simulink model "allen_var_test"  (R2018b)
settings: Solver=FixedStepAuto  StartTime=0.0  StopTime=10.0  FixedStep=simParams.sample_time_s  RelTol=1e-3
undefined symbols (not defined in the file or in its folder): fswParams, gyroscope_lib, simParams
libraries: simulink x3
settings Model: Creator=Taylor  LastModifiedBy=Taylor

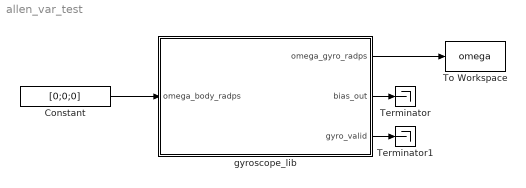
== system allen_var_test ==
  Constant : Constant  Value=[0;0;0]
  Terminator : Terminator
  Terminator1 : Terminator
  To Workspace : ToWorkspace  VariableName=omega  SampleTime=-1
      settings: Save2DSignal=2-D array (concatenate along first dimension)
  gyroscope_lib : Subsystem  AncestorBlock=gyroscope_lib/gyroscope_lib  mask{id_s=1}
      mask prompts: id_s "Choose the sensor ID"
      mask TypeOptions id_s: 1 | 2 | 3
      mask DialogControl DescGroupVar Prompt: SOC-i Gyroscope Model
      mask DialogControl DescTextVar Prompt: The spacecraft has three Bosch BMI055 gyroscopes.
  wires:
  Constant/1 -> gyroscope_lib/1(omega_body_radps)
  gyroscope_lib/1(omega_gyro_radps) -> To Workspace/1
  gyroscope_lib/2(bias_out) -> Terminator/1
  gyroscope_lib/3(gyro_valid) -> Terminator1/1

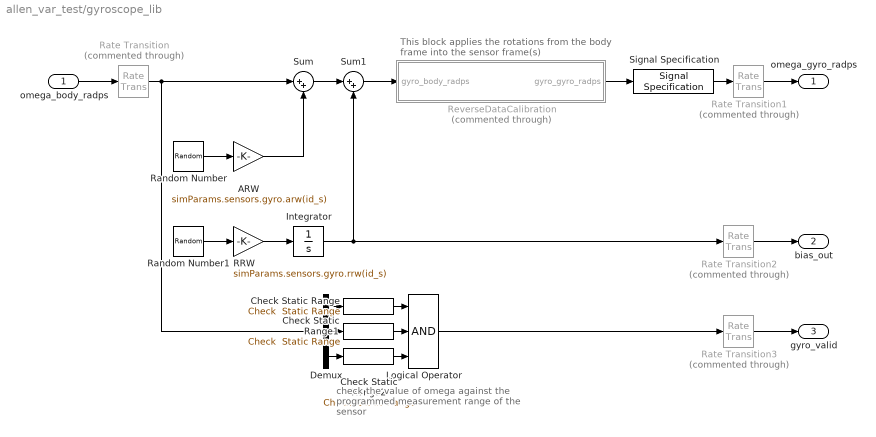
== system allen_var_test/gyroscope_lib ==
  note: check the value of omega against
      | the programmed measurement range
      | of the sensor
  note: This block applies the rotations from the
      | body frame into the sensor frame(s)
  omega_body_radps : Inport
  ARW : Gain  Gain=simParams.sensors.gyro.arw(id_s)
  Check Static Range : simulink/Model Verification/Check  Static Range  Description=simParams.sensors.gyro.w_min(id_s) <= u <= simParams.sensors.gyro.w_max(id_s)  max=simParams.sensors.gyro.w_max(id_s)  max_included=on  min=simParams.sensors.gyro.w_min(id_s)  min_included=on  enabled=on  stopWhenAssertionFail=off  export=on  icon=graphic
      settings: SourceProductName=Simulink  SourceProductBaseCode=SL
  Check Static Range1 : simulink/Model Verification/Check  Static Range  Description=simParams.sensors.gyro.w_min(id_s) <= u <= simParams.sensors.gyro.w_max(id_s)  max=simParams.sensors.gyro.w_max(id_s)  max_included=on  min=simParams.sensors.gyro.w_min(id_s)  min_included=on  enabled=on  stopWhenAssertionFail=off  export=on  icon=graphic
      settings: SourceProductName=Simulink  SourceProductBaseCode=SL
  Check Static Range2 : simulink/Model Verification/Check  Static Range  Description=simParams.sensors.gyro.w_min(id_s) <= u <= simParams.sensors.gyro.w_max(id_s)  max=simParams.sensors.gyro.w_max(id_s)  max_included=on  min=simParams.sensors.gyro.w_min(id_s)  min_included=on  enabled=on  stopWhenAssertionFail=off  export=on  icon=graphic
      settings: SourceProductName=Simulink  SourceProductBaseCode=SL
  Demux : Demux  Outputs=3
  Integrator : Integrator  InitialCondition=simParams.sensors.gyro.bias_init(:,id_s)
  Logical Operator : Logic  Inputs=3  AllPortsSameDT=off  OutDataTypeStr=boolean
  RRW : Gain  Gain=simParams.sensors.gyro.rrw(id_s)
  Random Number : RandomNumber  Mean=[0 0 0]  Variance=[1 1 1]  Seed=simParams.sensors.gyro.seed_arw(:,id_s)  SampleTime=simParams.sample_time_s
  Random Number1 : RandomNumber  Mean=[0 0 0]  Variance=[1 1 1]  Seed=simParams.sensors.gyro.seed_rrw(:,id_s)  SampleTime=simParams.sample_time_s
  Rate Transition : RateTransition  Commented=through  InitialCondition=simParams.initialConditions.w_body_radps  OutPortSampleTime=simParams.sensors.gyro.sample_time_s
  Rate Transition1 : RateTransition  Commented=through  InitialCondition=simParams.initialConditions.w_body_radps
  Rate Transition2 : RateTransition  Commented=through  InitialCondition=simParams.sensors.gyro.bias_init(id_s)
  Rate Transition3 : RateTransition  Commented=through  InitialCondition=1
  ReverseDataCalibration : Subsystem  Commented=through
  Signal Specification : SignalSpecification  Dimensions=3
  Sum : Sum  Inputs=|++
  Sum1 : Sum  Inputs=|++
  omega_gyro_radps : Outport
  bias_out : Outport  Port=2
  gyro_valid : Outport  Port=3
  wires:
  ReverseDataCalibration/1(gyro_gyro_radps) -> Signal Specification/1
  Sum1/1 -> ReverseDataCalibration/1(gyro_body_radps)
  Signal Specification/1 -> Rate Transition1/1
  Check Static Range2/1 -> Logical Operator/3
  Check Static Range/1 -> Logical Operator/1
  Check Static Range1/1 -> Logical Operator/2
  Demux/1 -> Check Static Range/1
  Demux/2 -> Check Static Range1/1
  Demux/3 -> Check Static Range2/1
  Rate Transition3/1 -> gyro_valid/1
  Rate Transition2/1 -> bias_out/1
  Rate Transition1/1 -> omega_gyro_radps/1
  Rate Transition/1 -> Sum/1, Demux/1
  ARW/1 -> Sum/2
  Integrator/1 -> Sum1/2, Rate Transition2/1
  Logical Operator/1 -> Rate Transition3/1
  RRW/1 -> Integrator/1
  Sum/1 -> Sum1/1
  omega_body_radps/1 -> Rate Transition/1
  Random Number1/1 -> RRW/1
  Random Number/1 -> ARW/1

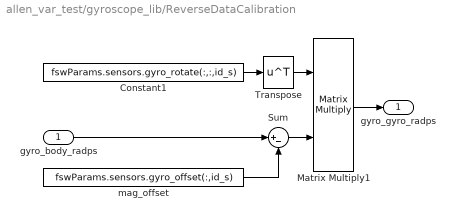
== system allen_var_test/gyroscope_lib/ReverseDataCalibration ==
  gyro_body_radps : Inport
  Constant1 : Constant  Value=fswParams.sensors.gyro_rotate(:,:,id_s)
  Matrix Multiply1 : Product  Multiplication=Matrix(*)
  Sum : Sum  Inputs=|+-
  Transpose : Math  Operator=transpose  SaturateOnIntegerOverflow=on
  mag_offset : Constant  Value=fswParams.sensors.gyro_offset(:,id_s)
  gyro_gyro_radps : Outport
  wires:
  mag_offset/1 -> Sum/2
  Sum/1 -> Matrix Multiply1/2
  gyro_body_radps/1 -> Sum/1
  Matrix Multiply1/1 -> gyro_gyro_radps/1
  Transpose/1 -> Matrix Multiply1/1
  Constant1/1 -> Transpose/1
